simulink model "SerialReader02"  (R2024a)
settings: Solver=ode4  StartTime=0.0  StopTime=tFinal_s  FixedStep=dt_s  RelTol=1e-3
values from neighbouring files (symbols this model uses):
  dt_s = 1    [MAIN_SerialReader02.m]
undefined symbols (not defined in the file or in its folder): LF
libraries: instrumentseriallib x2
settings Model: Creator=chris  LastModifiedBy=chris

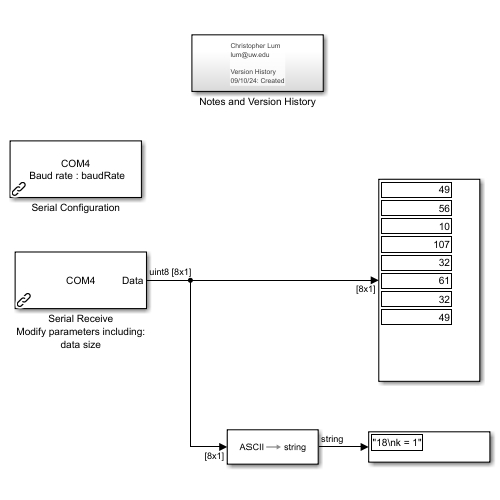
[thumbnail: Simulink's stored preview of the top-level diagram]
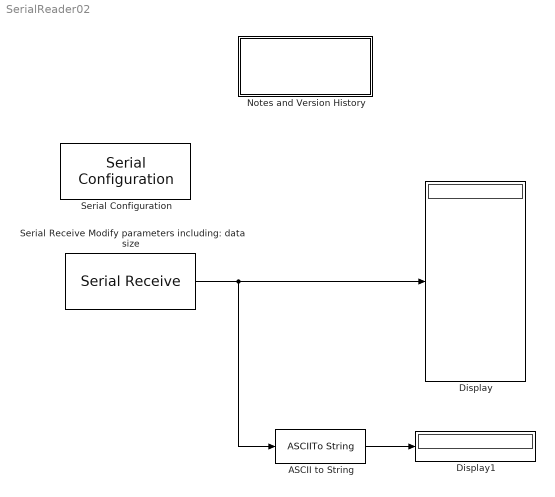
== system SerialReader02 ==
  ASCII to String : ASCIIToString
  Display : Display
  Display1 : Display
  Notes and Version History : Subsystem
  Serial Configuration : instrumentseriallib/Serial Configuration  Priority=-200000  PortSel=COM4  Port=COM4  ComPort=COM4  BaudRate=baudRate  DataBits=8  Parity=none  StopBits=1  ByteOrder=little-endian  FlowControl=none  Timeout=10  SimulateUsing=Interpreted execution  BlockInModel=on  aMode=1
  Serial Receive Modify parameters including: data size : instrumentseriallib/Serial Receive  Priority=1  PortSel=COM4  Port=COM4  ComPort=COM4  DataType=uint8  SaveDataType=uint8  ToggleHeader=off  Header=[]  ToggleDataSize=on  DataSize=serialReceive.dataSize  ToggleTerminator=off  Terminator=LF ('\n')  CustomTerminator=[]  InputFormat=Column major  EnableBlockingMode=on  ActionDataUnavailable=Output last received value  ActionWhenDataUnavailable=Output last received value  CustomValue=0  SampleTime=dt_s  SimulateUsing=Interpreted execution  BlockInModel=on  aMode=1
  wires:
  Serial Receive Modify parameters including: data size/1 -> ASCII to String/1, Display/1
  ASCII to String/1 -> Display1/1

== system SerialReader02/Notes and Version History ==
  note: Christopher Lum
      | lum@uw.edu
      |
      | Version History
      | 09/10/24: Created
